simulink model "moment_simulate"  (R2018a)
settings: Solver=FixedStepAuto  StartTime=0.0  StopTime=1000  FixedStep=dt  RelTol=1e-3
undefined symbols (not defined in the file or in its folder): dt, M_des
settings Model: Creator=Meng Chaoheng  LastModifiedBy=Meng Chaoheng

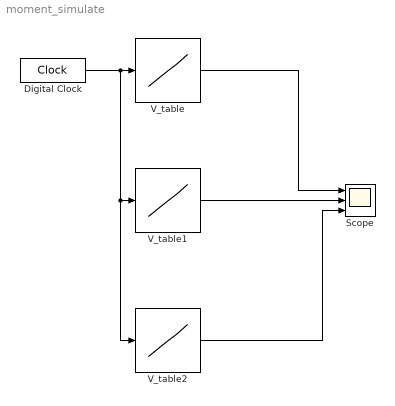
== system moment_simulate ==
  Digital Clock : DigitalClock  SampleTime=dt
  Scope : Scope  NumInputPorts=3
  V_table : Lookup  InputValues=t  Table=M_des(:,1)  LookUpMeth=Interpolation-Use End Values
  V_table1 : Lookup  InputValues=t  Table=M_des(:,2)  LookUpMeth=Interpolation-Use End Values
  V_table2 : Lookup  InputValues=t  Table=M_des(:,3)  LookUpMeth=Interpolation-Use End Values
  wires:
  Digital Clock/1 -> V_table1/1, V_table2/1, V_table/1
  V_table/1 -> Scope/1
  V_table1/1 -> Scope/2
  V_table2/1 -> Scope/3
